simulink subsystem "PieroCalculos"  (R2023b)
settings: Solver=VariableStepAuto  StartTime=0.0  StopTime=10.0  RelTol=1e-3
settings Model: Creator=Usuario  LastModifiedBy=Usuario

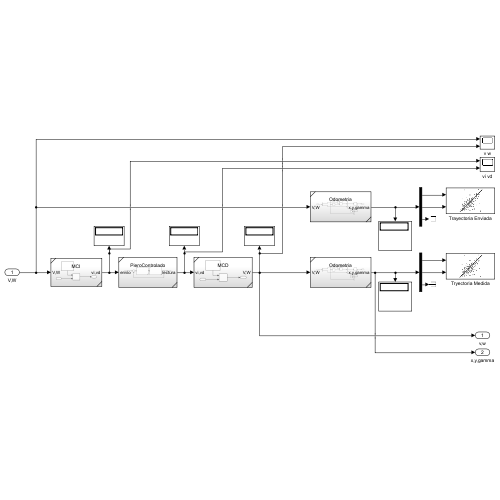
[thumbnail: Simulink's stored preview of the top-level diagram]
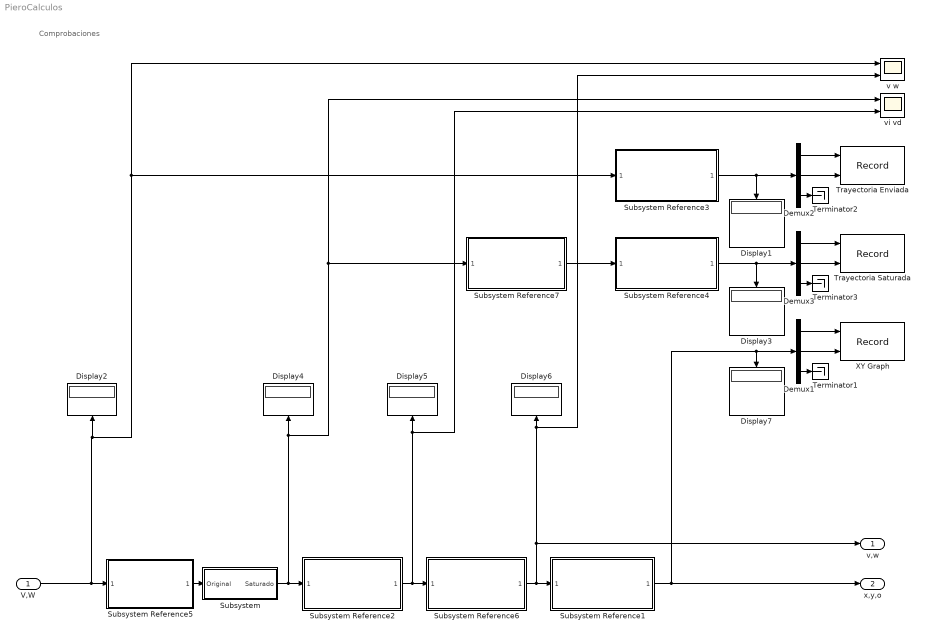
== system PieroCalculos ==
  note: Comprobaciones
  V,W : Inport
  Demux1 : Demux  Outputs=3
  Demux2 : Demux  Outputs=3
  Demux3 : Demux  Outputs=3
  Display{1..7} (7 alike) : Display
  Subsystem : Subsystem
  Subsystem Reference1 : Subsystem  ReferencedSubsystem=Odometria
  Subsystem Reference2 : Subsystem  ReferencedSubsystem=PieroControlado
  Subsystem Reference3 : Subsystem  ReferencedSubsystem=Odometria
  Subsystem Reference4 : Subsystem  ReferencedSubsystem=Odometria
  Subsystem Reference5 : Subsystem  ReferencedSubsystem=MCI
  Subsystem Reference6 : Subsystem  ReferencedSubsystem=MCD
  Subsystem Reference7 : Subsystem  ReferencedSubsystem=MCD
  Terminator1 : Terminator
  Terminator2 : Terminator
  Terminator3 : Terminator
  Trayectoria Enviada : Record  FileSettingsInternal="{\"entries\":[{\"content\":{\"excelSettings\":{\"content\":{},\"type\":\"Streamout.ExcelSettings\"}},\"type\":\"Streamout.FileSettingStorage\",\"uuid\":\"\"}],\"packageUris\":[\"http:\\/\\/schema.mathworks.com\\/mf0\\/streamout_blocks\\/R2020a\"],\"version\":\"1.0\"}"  Layout=[1 1]  SignalsInternal="{\"entries\":[{\"content\":{\"signals\":[{\"content\":{\"blockPath\":[],\"dimensions\":[1],\"domain\":\"\",\"lineColor\":\"#a2142f\",\"plots\":[ 1 ],\"port\":1,\"signalID\":1,\"signalName\":\"XY Graph:1\"},\"type\":\"RecordBlkView.Signal\",\"uuid\":\"\"},{\"content\":{\"blockPath\":[],\"dimensions\":[1],\"domain\":\"\",\"lineColor\":\"#139fff\",\"plots\":[ 1 ],\"port\":2,\"signalID\":2,\"signalName\":\"XY Graph:2\"},\"type\":\"RecordBlkView.Signal\",\"uuid\":\"\"}]},\"type\":\"RecordBlkView.InputSignals\",\"uuid\":\"\"}],\"packageUris\":[\"http:\\/\\/schema.mathworks.com\\/mf0\\/streamout_blocks\\/R2020a\"],\"version\":\"1.0\"}"  VisualizationBindings="{\"xyplotplugin\":{\"info\":[{\"series\":[{\"bindingParametersList\":[{\"parameter\":\"X-Axis\",\"signalID\":1,\"signalName\":\"XY Graph:1\"},{\"parameter\":\"Y-Axis\",\"signalID\":2,\"signalName\":\"XY Graph:2\"}],\"seriesID\":0}],\"subplotID\":1}]}}"  CompatibilityTag=XY
  Trayectoria Saturada : Record  FileSettingsInternal="{\"entries\":[{\"content\":{\"excelSettings\":{\"content\":{},\"type\":\"Streamout.ExcelSettings\"}},\"type\":\"Streamout.FileSettingStorage\",\"uuid\":\"\"}],\"packageUris\":[\"http:\\/\\/schema.mathworks.com\\/mf0\\/streamout_blocks\\/R2020a\"],\"version\":\"1.0\"}"  Layout=[1 1]  SignalsInternal="{\"entries\":[{\"content\":{\"signals\":[{\"content\":{\"blockPath\":[],\"dimensions\":[1],\"domain\":\"\",\"lineColor\":\"#a2142f\",\"plots\":[ 1 ],\"port\":1,\"signalID\":1,\"signalName\":\"XY Graph:1\"},\"type\":\"RecordBlkView.Signal\",\"uuid\":\"\"},{\"content\":{\"blockPath\":[],\"dimensions\":[1],\"domain\":\"\",\"lineColor\":\"#139fff\",\"plots\":[ 1 ],\"port\":2,\"signalID\":2,\"signalName\":\"XY Graph:2\"},\"type\":\"RecordBlkView.Signal\",\"uuid\":\"\"}]},\"type\":\"RecordBlkView.InputSignals\",\"uuid\":\"\"}],\"packageUris\":[\"http:\\/\\/schema.mathworks.com\\/mf0\\/streamout_blocks\\/R2020a\"],\"version\":\"1.0\"}"  VisualizationBindings="{\"xyplotplugin\":{\"info\":[{\"series\":[{\"bindingParametersList\":[{\"parameter\":\"X-Axis\",\"signalID\":1,\"signalName\":\"XY Graph:1\"},{\"parameter\":\"Y-Axis\",\"signalID\":2,\"signalName\":\"XY Graph:2\"}],\"seriesID\":0}],\"subplotID\":1}]}}"  CompatibilityTag=XY
  XY Graph : Record  FileSettingsInternal="{\"entries\":[{\"content\":{\"excelSettings\":{\"content\":{},\"type\":\"Streamout.ExcelSettings\"}},\"type\":\"Streamout.FileSettingStorage\",\"uuid\":\"\"}],\"packageUris\":[\"http:\\/\\/schema.mathworks.com\\/mf0\\/streamout_blocks\\/R2020a\"],\"version\":\"1.0\"}"  Layout=[1 1]  SignalsInternal="{\"entries\":[{\"content\":{\"signals\":[{\"content\":{\"blockPath\":[],\"dimensions\":[1],\"domain\":\"\",\"lineColor\":\"#a2142f\",\"plots\":[ 1 ],\"port\":1,\"signalID\":1,\"signalName\":\"Demux1:1\"},\"type\":\"RecordBlkView.Signal\",\"uuid\":\"\"},{\"content\":{\"blockPath\":[],\"dimensions\":[1],\"domain\":\"\",\"lineColor\":\"#139fff\",\"plots\":[ 1 ],\"port\":2,\"signalID\":2,\"signalName\":\"Demux1:2\"},\"type\":\"RecordBlkView.Signal\",\"uuid\":\"\"}]},\"type\":\"RecordBlkView.InputSignals\",\"uuid\":\"\"}],\"packageUris\":[\"http:\\/\\/schema.mathworks.com\\/mf0\\/streamout_blocks\\/R2020a\"],\"version\":\"1.0\"}"  VisualizationBindings="{\"xyplotplugin\":{\"info\":[{\"series\":[{\"bindingParametersList\":[{\"parameter\":\"X-Axis\",\"signalID\":1,\"signalName\":\"Demux1:1\"},{\"parameter\":\"Y-Axis\",\"signalID\":2,\"signalName\":\"Demux1:2\"}],\"seriesID\":0}],\"subplotID\":1}]}}"  CompatibilityTag=XY
  v w : Scope  NumInputPorts=2
  vi vd : Scope  NumInputPorts=2
  v,w : Outport
  x,y,o : Outport  Port=2
  wires:
  Demux2/3 -> Terminator2/1
  Subsystem Reference3/1 -> Demux2/1, Display1/1
  Demux1/2 -> XY Graph/2
  Demux2/2 -> Trayectoria Enviada/2
  Subsystem Reference6/1 -> Subsystem Reference1/1, v,w/1, v w/2, Display6/1
  Demux1/1 -> XY Graph/1
  Demux1/3 -> Terminator1/1
  Subsystem Reference1/1 -> Demux1/1, Display7/1, x,y,o/1
  Subsystem Reference2/1 -> Subsystem Reference6/1, vi vd/2, Display5/1
  Demux2/1 -> Trayectoria Enviada/1
  V,W/1 -> Subsystem Reference3/1, v w/1, Display2/1, Subsystem Reference5/1
  Demux3/1 -> Trayectoria Saturada/1
  Demux3/3 -> Terminator3/1
  Demux3/2 -> Trayectoria Saturada/2
  Subsystem Reference4/1 -> Demux3/1, Display3/1
  Subsystem Reference7/1 -> Subsystem Reference4/1
  Subsystem/1(Saturado) -> Subsystem Reference2/1, vi vd/1, Subsystem Reference7/1, Display4/1
  Subsystem Reference5/1 -> Subsystem/1(Original)

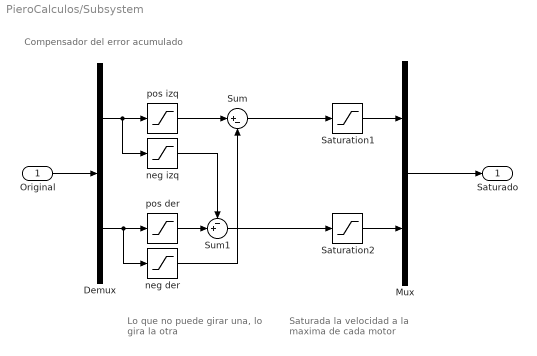
== system PieroCalculos/Subsystem ==
  note: Compensador del error acumulado
  note: Lo que no puede girar una,
      | lo gira la otra
  note: Saturada la velocidad a la
      | maxima de cada motor
  Original : Inport
  Demux : Demux  Outputs=2
  Mux : Mux  Inputs=2
  Saturation1 : Saturate  UpperLimit=0.4883  LowerLimit=0
  Saturation2 : Saturate  UpperLimit=0.4811  LowerLimit=0
  Sum : Sum  Inputs=|+-
  Sum1 : Sum  Inputs=-+|
  neg der : Saturate  UpperLimit=0  LowerLimit=-inf
  neg izq : Saturate  UpperLimit=0  LowerLimit=-inf
  pos der : Saturate  UpperLimit=inf  LowerLimit=0
  pos izq : Saturate  UpperLimit=inf  LowerLimit=0
  Saturado : Outport
  wires:
  Saturation2/1 -> Mux/2
  Saturation1/1 -> Mux/1
  Mux/1 -> Saturado/1
  neg der/1 -> Sum/2
  neg izq/1 -> Sum1/1
  Demux/2 -> pos der/1, neg der/1
  Demux/1 -> pos izq/1, neg izq/1
  Sum1/1 -> Saturation2/1
  pos izq/1 -> Sum/1
  Sum/1 -> Saturation1/1
  pos der/1 -> Sum1/2
  Original/1 -> Demux/1
